simulink model "ap_12BAdapted_with_contracts_AutoPilot"  (R2017b)
settings: Solver=FixedStepDiscrete  StartTime=0.0  StopTime=500  FixedStep=Ts  RelTol=1e-3  EnableMultiTasking=on
undefined symbols (not defined in the file): beaver_b, beaver_c, beaver_mass, beaver_S, Cl0, Cl_alpha2_dpt, Cl_beta, Cl_da, Cl_da_alpha, Cl_dr, Cl_p, Cl_r, Cm0, Cm_alpha, Cm_alpha2, Cm_beta2, Cm_de, Cm_df, Cm_dpt, Cm_q, Cm_r, Cn0, Cn_beta, Cn_beta3, Cn_da, Cn_dpt3, Cn_dr, Cn_p, Cn_q, Cn_r, contractAfterSimulation, contractBeforeSimulation, ContractBlock, ContractEnsureBlock, ContractGuaranteeBlock, ContractModeBlock, ContractRequireBlock, ContractValidatorBlock, Cx0, Cx_alpha, Cx_alpha2, Cx_alpha3, Cx_df, Cx_df_alpha, Cx_dpt, Cx_dpt2_alpha, Cx_dr, Cx_q, Cy0, Cy_beta, Cy_da, Cy_dr, Cy_dr_alpha, Cy_p, Cy_r, Cz0, Cz_alpha, Cz_alpha3, Cz_de, Cz_de_beta ... (+32)
libraries: simulink x10, cocosimLibs x3
(part 1 of 4)
settings Model: Creator=elliocm  LastModifiedBy=hbourbou
settings DataIOCC: LimitDataPoints=on  SaveFormat=Array
settings OptimizationCC: ExpressionDepthLimit=2147483647  LifeSpan=inf
settings DebuggingCC: SolverPrmCheckMsg=warning  StateNameClashWarn=warning  SFUnexpectedBacktrackingDiag=warning  SFNoUnconditionalDefaultTransitionDiag=warning  SFExecutionAtInitializationDiag=none
settings HardwareCC: ProdBitPerPointer=32  ProdBitPerSizeT=32  ProdBitPerPtrDiffT=32  ProdLargestAtomicFloat=None  ProdIntDivRoundTo=Undefined  ProdEndianess=Unspecified  ProdWordSize=32  ProdHWDeviceType=32-bit Generic
settings ModelReferenceCC: PropagateSignalLabelsOutOfModel=off
settings CodeAppCC: StateflowObjectComments=on
settings GRTTargetCC: TargetLangStandard=C89/C90 (ANSI)  GeneratePreprocessorConditionals=Disable all
settings ConfigComp: CovMetricSettings=dw  CovHtmlReporting=on  CovSaveCumulativeToWorkspaceVar=on  CovSaveSingleToWorkspaceVar=on  CovExternalEMLEnable=off

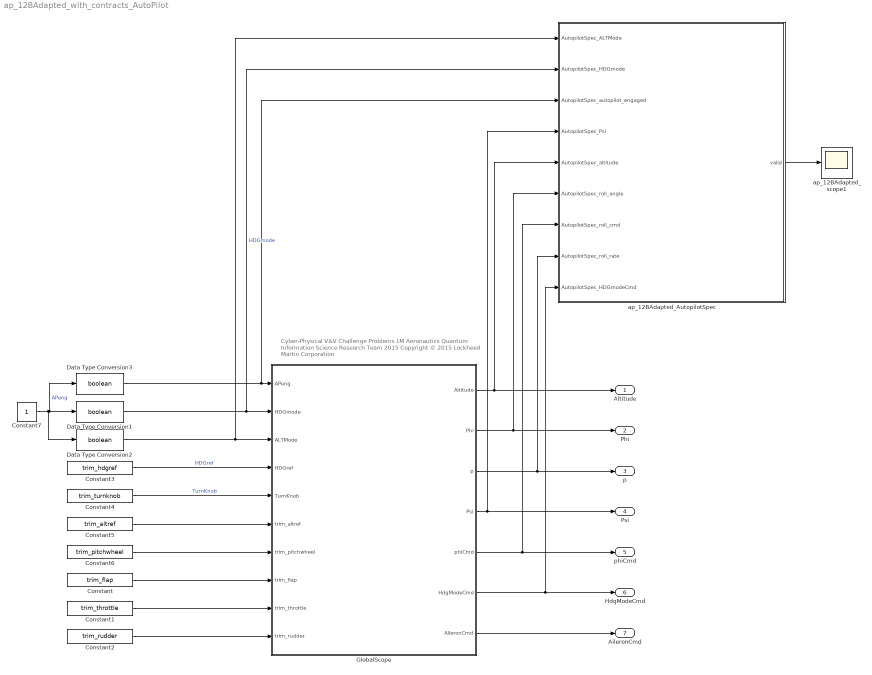
== system ap_12BAdapted_with_contracts_AutoPilot ==
  note: Cyber-Physical V&V Challenge Problems
      | LM Aeronautics Quantum Information Science Research Team 2015
      | Copyright © 2015 Lockheed Martin Corporation
  Constant : Constant  Value=trim_flap
  Constant1 : Constant  Value=trim_throttle
  Constant2 : Constant  Value=trim_rudder
  Constant3 : Constant  Value=trim_hdgref
  Constant4 : Constant  Value=trim_turnknob
  Constant5 : Constant  Value=trim_altref
  Constant6 : Constant  Value=trim_pitchwheel
  Constant7 : Constant
  Data Type Conversion1 : DataTypeConversion  OutDataTypeStr=boolean
  Data Type Conversion2 : DataTypeConversion  OutDataTypeStr=boolean
  Data Type Conversion3 : DataTypeConversion  OutDataTypeStr=boolean
  GlobalScope : Subsystem
  ap_12BAdapted_AutopilotSpec : Subsystem  mask(ContractBlock){ContractBlockType=ContractBlock}
      mask init:
      | set_param(gcb, 'LinkStatus', 'none');
      mask DialogControl DescTextVar Prompt: Contract block
      mask Display:
      | text(0.5, 0.5, '{\bf\fontsize{20}Contract}', 'hor', 'center', 'texmode','on');
      | blocks = find_system(gcb, 'LookUnderMasks','all', 'SearchDepth',1,'BlockType','Inport');
      | for i = 1 : length(blocks)
      |     blockName = get_param(blocks(i), 'Name');
      |     [path, blockName] = fileparts(char(blockName));
      |     port_label('input', i, blockName);
      | end
      | 
      | blocks = find_system(gcb, 'LookUnderMasks','all', 'SearchDepth',1,'BlockType','Outport');
      | for i = 1 : length(blocks)
      |     blockName = get_param(blocks(i), 'Name');
      |     [path, blockName] = fileparts(char(blockName));
      |     port_label('output', i, blockName);
      | end
  ap_12BAdapted_scope1 : Scope
  Altitude : Outport  VectorParamsAs1DForOutWhenUnconnected=off
  Phi : Outport  Port=2  VectorParamsAs1DForOutWhenUnconnected=off
  p : Outport  Port=3  VectorParamsAs1DForOutWhenUnconnected=off
  Psi : Outport  Port=4  VectorParamsAs1DForOutWhenUnconnected=off
  phiCmd : Outport  Port=5  VectorParamsAs1DForOutWhenUnconnected=off
  HdgModeCmd : Outport  Port=6  VectorParamsAs1DForOutWhenUnconnected=off
  AileronCmd : Outport  Port=7  VectorParamsAs1DForOutWhenUnconnected=off
  wires:
  Constant7/1 -> Data Type Conversion2/1, Data Type Conversion3/1, Data Type Conversion1/1  "APeng"
  Data Type Conversion3/1 -> ap_12BAdapted_AutopilotSpec/3(AutopilotSpec_autopilot_engaged), GlobalScope/1(APeng)
  Data Type Conversion1/1 -> ap_12BAdapted_AutopilotSpec/2(AutopilotSpec_HDGmode), GlobalScope/2(HDGmode)  "HDGmode"
  Data Type Conversion2/1 -> ap_12BAdapted_AutopilotSpec/1(AutopilotSpec_ALTMode), GlobalScope/3(ALTMode)
  Constant3/1 -> GlobalScope/4(HDGref)  "HDGref"
  Constant4/1 -> GlobalScope/5(TurnKnob)  "TurnKnob"
  Constant5/1 -> GlobalScope/6(trim_altref)
  Constant6/1 -> GlobalScope/7(trim_pitchwheel)
  GlobalScope/1(Altitude) -> ap_12BAdapted_AutopilotSpec/5(AutopilotSpec_altitude), Altitude/1
  Constant/1 -> GlobalScope/8(trim_flap)
  Constant2/1 -> GlobalScope/10(trim_rudder)
  Constant1/1 -> GlobalScope/9(trim_throttle)
  GlobalScope/6(HdgModeCmd) -> ap_12BAdapted_AutopilotSpec/9(AutopilotSpec_HDGmodeCmd), HdgModeCmd/1
  GlobalScope/5(phiCmd) -> ap_12BAdapted_AutopilotSpec/7(AutopilotSpec_roll_cmd), phiCmd/1
  GlobalScope/7(AileronCmd) -> AileronCmd/1
  GlobalScope/4(Psi) -> ap_12BAdapted_AutopilotSpec/4(AutopilotSpec_Psi), Psi/1
  GlobalScope/3(p) -> ap_12BAdapted_AutopilotSpec/8(AutopilotSpec_roll_rate), p/1
  GlobalScope/2(Phi) -> ap_12BAdapted_AutopilotSpec/6(AutopilotSpec_roll_angle), Phi/1
  ap_12BAdapted_AutopilotSpec/1(valid) -> ap_12BAdapted_scope1/1

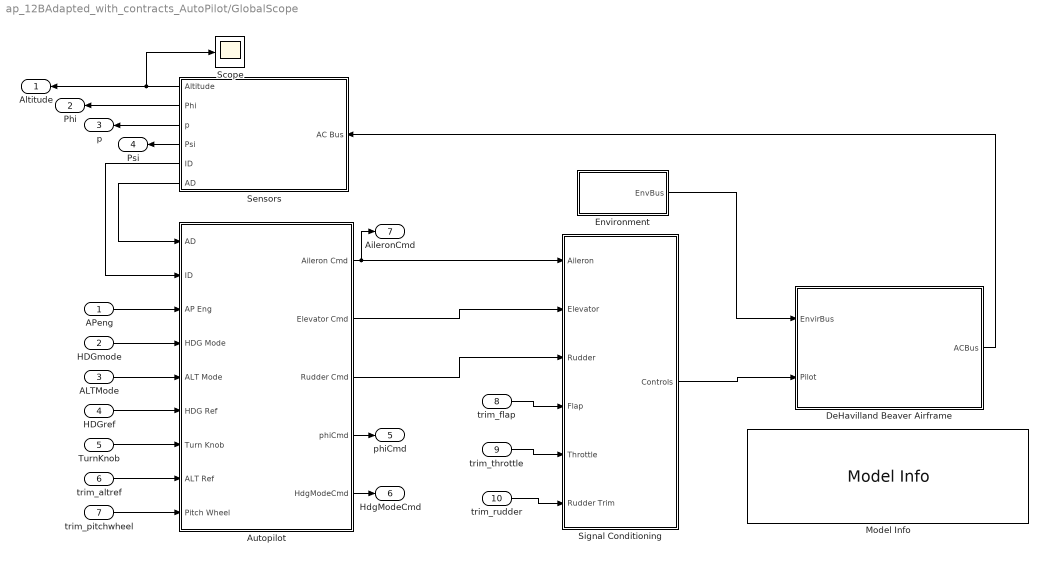
== system ap_12BAdapted_with_contracts_AutoPilot/GlobalScope ==
  APeng : Inport
  HDGmode : Inport  Port=2
  ALTMode : Inport  Port=3
  HDGref : Inport  Port=4
  TurnKnob : Inport  Port=5
  trim_altref : Inport  Port=6
  trim_pitchwheel : Inport  Port=7
  trim_flap : Inport  Port=8
  trim_throttle : Inport  Port=9
  trim_rudder : Inport  Port=10
  Autopilot : Subsystem  TreatAsAtomicUnit=on
  DeHavilland Beaver Airframe : Subsystem  TreatAsAtomicUnit=on
      mask Display:
      | %image(imread('asbbeaver.jpg'))
      | image(imread('asbbeaver.png'))
  Environment : Subsystem
  Model Info : simulink/Model-Wide Utilities/Model Info  Frame=on  DisplayStringWithTags=|  HorizontalTextAlignment=Center  LeftAlignmentValue=0.5
      | DeHavilland Beaver model 
      | originally based on work created by
      | Marc Rauw for Delft University of Technology,  
      | http://www.dutchroll.com
      | and subsequently modified by the Mathworks
      | http://www.mathworks.com/matlabcentral/fileexchange/
  Scope : Scope
  Sensors : Subsystem
  Signal Conditioning : Subsystem  TreatAsAtomicUnit=on
  Altitude : Outport  VectorParamsAs1DForOutWhenUnconnected=off
  Phi : Outport  Port=2  VectorParamsAs1DForOutWhenUnconnected=off
  p : Outport  Port=3  VectorParamsAs1DForOutWhenUnconnected=off
  Psi : Outport  Port=4  VectorParamsAs1DForOutWhenUnconnected=off
  phiCmd : Outport  Port=5  VectorParamsAs1DForOutWhenUnconnected=off
  HdgModeCmd : Outport  Port=6  VectorParamsAs1DForOutWhenUnconnected=off
  AileronCmd : Outport  Port=7  VectorParamsAs1DForOutWhenUnconnected=off
  wires:
  Autopilot/1(Aileron Cmd) -> AileronCmd/1, Signal Conditioning/1(Aileron)
  Sensors/1(Altitude) -> Altitude/1, Scope/1
  trim_altref/1 -> Autopilot/8(ALT Ref)
  Autopilot/3(Rudder Cmd) -> Signal Conditioning/3(Rudder)
  ALTMode/1 -> Autopilot/5(ALT Mode)
  TurnKnob/1 -> Autopilot/7(Turn Knob)
  trim_throttle/1 -> Signal Conditioning/5(Throttle)
  trim_rudder/1 -> Signal Conditioning/6(Rudder Trim)
  trim_flap/1 -> Signal Conditioning/4(Flap)
  trim_pitchwheel/1 -> Autopilot/9(Pitch Wheel)
  APeng/1 -> Autopilot/3(AP Eng)
  Environment/1(EnvBus) -> DeHavilland Beaver Airframe/1(EnvirBus)
  Autopilot/2(Elevator Cmd) -> Signal Conditioning/2(Elevator)
  DeHavilland Beaver Airframe/1(ACBus) -> Sensors/1(AC Bus)
  HDGmode/1 -> Autopilot/4(HDG Mode)
  HDGref/1 -> Autopilot/6(HDG Ref)
  Sensors/6(AD) -> Autopilot/1(AD)
  Sensors/5(ID) -> Autopilot/2(ID)
  Autopilot/4(phiCmd) -> phiCmd/1
  Sensors/2(Phi) -> Phi/1
  Sensors/3(p) -> p/1
  Autopilot/5(HdgModeCmd) -> HdgModeCmd/1
  Sensors/4(Psi) -> Psi/1
  Signal Conditioning/1(Controls) -> DeHavilland Beaver Airframe/2(Pilot)

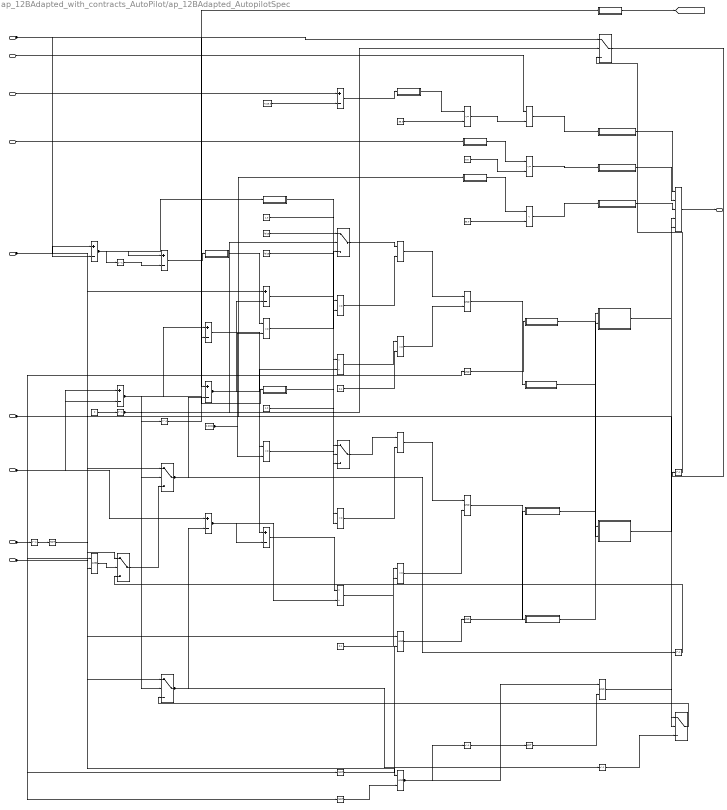
== system ap_12BAdapted_with_contracts_AutoPilot/ap_12BAdapted_AutopilotSpec ==
  AutopilotSpec_ALTMode : Inport  OutDataTypeStr=boolean
  AutopilotSpec_HDGmode : Inport  Port=2  OutDataTypeStr=boolean
  AutopilotSpec_autopilot_engaged : Inport  Port=3  OutDataTypeStr=boolean
  AutopilotSpec_Psi : Inport  Port=4  OutDataTypeStr=double
  AutopilotSpec_altitude : Inport  Port=5  OutDataTypeStr=double
  AutopilotSpec_roll_angle : Inport  Port=6  OutDataTypeStr=double
  AutopilotSpec_roll_cmd : Inport  Port=7  OutDataTypeStr=double
  AutopilotSpec_roll_rate : Inport  Port=8  OutDataTypeStr=double
  AutopilotSpec_HDGmodeCmd : Inport  Port=9  OutDataTypeStr=double
  AP-000 : Subsystem  mask(ContractGuaranteeBlock){ContractBlockType=ContractGuaranteeBlock}
      mask init:
      | set_param(gcb, 'LinkStatus', 'none');
      mask DialogControl DescTextVar Prompt: Guarantee block
  AP-005 : Subsystem  mask(ContractGuaranteeBlock){ContractBlockType=ContractGuaranteeBlock}
      mask init:
      | set_param(gcb, 'LinkStatus', 'none');
      mask DialogControl DescTextVar Prompt: Guarantee block
  AP-006 : Subsystem  mask(ContractGuaranteeBlock){ContractBlockType=ContractGuaranteeBlock}
      mask init:
      | set_param(gcb, 'LinkStatus', 'none');
      mask DialogControl DescTextVar Prompt: Guarantee block
  Arrow_xxAutopilotSpec_9_ni_0 : Delay  DelayLength=1  InitialCondition=1
  PRE_xxAutopilotSpec_{10,13,16,20,25,28,31} (7 alike) : Delay  DelayLength=1  InitialCondition=0
  abs_real_call : Subsystem
  abs_real_call1 : Subsystem
  abs_real_call11 : Subsystem
  abs_real_call111 : Subsystem
  abs_real_call1111 : Subsystem
  abs_real_call11111 : Subsystem
  abs_real_call111111 : Subsystem
  branch_10_IF : Switch  Criteria=u2 ~= 0
  branch_11_IF : Switch  Criteria=u2 ~= 0
  branch_12_IF : Switch  Criteria=u2 ~= 0
  branch_13_IF : Switch  Criteria=u2 ~= 0
  branch_14_IF : Switch  Criteria=u2 ~= 0
  branch_15_IF : Switch  Criteria=u2 ~= 0
  branch_9_IF : Switch  Criteria=u2 ~= 0
  hdg_err_operator : Sum  Inputs=+-  OutDataTypeStr=double
  hdg_mode : Subsystem  mask(ContractModeBlock){ContractBlockType=ContractModeBlock}
      mask init:
      | set_param(gcb, 'LinkStatus', 'none');
      mask DialogControl DescTextVar Prompt: Mode block
  hdg_mode_ensure : Subsystem  mask(ContractEnsureBlock){ContractBlockType=ContractEnsureBlock}
      mask init:
      | set_param(gcb, 'LinkStatus', 'none');
      mask DialogControl DescTextVar Prompt: Ensure block
  hdg_mode_ensure_cond : Logic  AllPortsSameDT=off  OutDataTypeStr=boolean
  hdg_mode_require : Subsystem  mask(ContractRequireBlock){ContractBlockType=ContractRequireBlock}
      mask init:
      | set_param(gcb, 'LinkStatus', 'none');
      mask DialogControl DescTextVar Prompt: Require block
  hdg_mode_require_cond : Logic  Inputs=1  AllPortsSameDT=off  OutDataTypeStr=boolean
  hdg_overshoot_operator : Product  Inputs=*/  OutDataTypeStr=double
  hdg_step_operator : Sum  Inputs=+-  OutDataTypeStr=double
  overshoot_operator : Product  Inputs=*/  OutDataTypeStr=double
  rollHoldMode_operator : Logic  AllPortsSameDT=off  OutDataTypeStr=boolean
  roll_err_operator : Sum  Inputs=+-  OutDataTypeStr=double
  roll_hold_mode : Subsystem  mask(ContractModeBlock){ContractBlockType=ContractModeBlock}
      mask init:
      | set_param(gcb, 'LinkStatus', 'none');
      mask DialogControl DescTextVar Prompt: Mode block
  roll_hold_mode_ensure : Subsystem  mask(ContractEnsureBlock){ContractBlockType=ContractEnsureBlock}
      mask init:
      | set_param(gcb, 'LinkStatus', 'none');
      mask DialogControl DescTextVar Prompt: Ensure block
  roll_hold_mode_ensure_cond : Logic  AllPortsSameDT=off  OutDataTypeStr=boolean
  roll_hold_mode_require : Subsystem  mask(ContractRequireBlock){ContractBlockType=ContractRequireBlock}
      mask init:
      | set_param(gcb, 'LinkStatus', 'none');
      mask DialogControl DescTextVar Prompt: Require block
  roll_hold_mode_require_cond : Logic  Inputs=1  AllPortsSameDT=off  OutDataTypeStr=boolean
  spec219_operator : Logic  AllPortsSameDT=off  OutDataTypeStr=boolean
  spec228_operator : cocosimLibs/Implies  SystemSampleTime=-1  Latency=0  AutoFrameSizeCalculation=off
  spec233_operator : RelationalOperator  Operator=<=  OutDataTypeStr=boolean  RndMeth=Simplest
  spec233_rhs_2 : Constant  Value=0.1  OutDataTypeStr=double
  spec244_operator : cocosimLibs/Implies  SystemSampleTime=-1  Latency=0  AutoFrameSizeCalculation=off
  spec249_operator : RelationalOperator  Operator=<=  OutDataTypeStr=boolean  RndMeth=Simplest
  spec249_rhs_2 : Constant  Value=0.1  OutDataTypeStr=double
  spec263_operator : cocosimLibs/Implies  SystemSampleTime=-1  Latency=0  AutoFrameSizeCalculation=off
  spec268_operator : RelationalOperator  Operator=<=  OutDataTypeStr=boolean  RndMeth=Simplest
  spec268_rhs_2 : Constant  Value=6.6  OutDataTypeStr=double
  spec273_operator : RelationalOperator  Operator=<  OutDataTypeStr=boolean  RndMeth=Simplest
  spec273_rhs_2 : Constant  Value=33.0  OutDataTypeStr=double
  step_operator : Sum  Inputs=+-  OutDataTypeStr=double
  validator : M-S-Function  LoadFcn=saveValidatorParameters(gcb);  InitFcn=contractBeforeSimulation();  StopFcn=contractAfterSimulation();  FunctionName=contract  mask(ContractValidatorBlock){assumePorts=0, guaranteePorts=3, modePorts=2, ContractBlockType=ContractValidatorBlock, createInportsCheckbox=off}
      mask prompts: assumePorts "Assume ports     :"; guaranteePorts "Guarantee ports :"; modePorts "Mode ports        :"; createInportsCheckbox "Create inports and connect them automatically"
      mask init:
      | set_param(gcb,'LinkStatus','none');
      | contract_callback('inputs_callback',gcb);
      mask DialogControl DescTextVar Prompt: The validator block implements the following logic: <br> <br> <b>Sofar</b>(assume<sub>1</sub> <b>&#8743;</b> assume<sub>2</sub> <b>&#8743;</b> ... assume<sub>k</sub>) <b>&rarr;</b> (guarantee<sub>1</sub> <b>&#8743;</b> guarantee<sub>2</sub> <b>&#8743;</b> ... guarantee<sub>m</sub> <b>&#8743;</b>  mode<sub>1</sub> <b>&#8743;</b> mode<sub>2</sub> <b>&#8743;</b> ... <b>&#8743;</b> mode<sub>n</sub> )<br> where mode<sub>i</sub> = require<sub>i</sub> <b>&rarr;</b> ensure<sub>i</sub>
      mask Display:
      | color('black');
      | port_label('input',1,'guarantee');
      | port_label('input',2,'guarantee');
      | port_label('input',3,'guarantee');
      | port_label('input',4,'mode');
      | port_label('input',5,'mode');
      | port_label('output',1,'valid');
  xxAutopilotSpec_11_operator : Logic  Operator=NOT  AllPortsSameDT=off  OutDataTypeStr=boolean
  xxAutopilotSpec_12_operator : Logic  AllPortsSameDT=off  OutDataTypeStr=boolean
  xxAutopilotSpec_15_operator : Logic  Operator=NOT  AllPortsSameDT=off  OutDataTypeStr=boolean
  xxAutopilotSpec_17_operator : Sum  Inputs=+-  OutDataTypeStr=double
  xxAutopilotSpec_18_operator : RelationalOperator  Operator=<=  OutDataTypeStr=boolean  RndMeth=Simplest
  xxAutopilotSpec_19_rhs1 : Constant  Value=false  OutDataTypeStr=boolean
  xxAutopilotSpec_1_operator : RelationalOperator  Operator=<=  OutDataTypeStr=boolean  RndMeth=Simplest
  xxAutopilotSpec_1_rhs_2 : Constant  Value=35.0  OutDataTypeStr=double
  xxAutopilotSpec_21_operator : Sum  Inputs=+-  OutDataTypeStr=double
  xxAutopilotSpec_23_operator : RelationalOperator  Operator=<=  OutDataTypeStr=boolean  RndMeth=Simplest
  xxAutopilotSpec_24_rhs1 : Constant  Value=false  OutDataTypeStr=boolean
  xxAutopilotSpec_27_operator : Sum  Inputs=+-  OutDataTypeStr=double
  xxAutopilotSpec_29_operator : Logic  Operator=NOT  AllPortsSameDT=off  OutDataTypeStr=boolean
  xxAutopilotSpec_30_operator : Logic  AllPortsSameDT=off  OutDataTypeStr=boolean
  xxAutopilotSpec_33_rhs : Constant  Value=7225.0  OutDataTypeStr=double
  xxAutopilotSpec_34_operator : Sum  Inputs=+-  OutDataTypeStr=double
  xxAutopilotSpec_3_operator : RelationalOperator  Operator=<=  OutDataTypeStr=boolean  RndMeth=Simplest
  xxAutopilotSpec_3_rhs_2 : Constant  Value=1.0  OutDataTypeStr=double
  xxAutopilotSpec_4_operator : Logic  Operator=NOT  AllPortsSameDT=off  OutDataTypeStr=boolean
  xxAutopilotSpec_6_operator : RelationalOperator  Operator=<=  OutDataTypeStr=boolean  RndMeth=Simplest
  xxAutopilotSpec_6_rhs_2 : Constant  Value=1.0  OutDataTypeStr=double
  xxAutopilotSpec_7_rhs : Constant  Value=0.0001  OutDataTypeStr=double
  xxAutopilotSpec_8_operator : Sum  Inputs=+-  OutDataTypeStr=double
  xxAutopilotSpec_9_ni_0_init : Constant  Value=0  OutDataTypeStr=boolean
  valid : Outport
  wires:
  validator/1 -> valid/1
  xxAutopilotSpec_6_rhs_2/1 -> xxAutopilotSpec_6_operator/2
  abs_real_call11111/1(abs_real_y) -> xxAutopilotSpec_6_operator/1
  xxAutopilotSpec_3_rhs_2/1 -> xxAutopilotSpec_3_operator/2
  abs_real_call1111/1(abs_real_y) -> xxAutopilotSpec_3_operator/1
  xxAutopilotSpec_33_rhs/1 -> xxAutopilotSpec_34_operator/2
  AutopilotSpec_altitude/1 -> xxAutopilotSpec_34_operator/1
  xxAutopilotSpec_29_operator/1 -> xxAutopilotSpec_30_operator/2
  PRE_xxAutopilotSpec_28/1 -> xxAutopilotSpec_29_operator/1
  abs_real_call111/1(abs_real_y) -> xxAutopilotSpec_23_operator/1
  PRE_xxAutopilotSpec_20/1 -> xxAutopilotSpec_21_operator/2
  xxAutopilotSpec_1_rhs_2/1 -> xxAutopilotSpec_1_operator/2
  abs_real_call11/1(abs_real_y) -> xxAutopilotSpec_1_operator/1
  xxAutopilotSpec_17_operator/1 -> xxAutopilotSpec_18_operator/1
  PRE_xxAutopilotSpec_16/1 -> xxAutopilotSpec_17_operator/2
  xxAutopilotSpec_11_operator/1 -> xxAutopilotSpec_12_operator/2
  PRE_xxAutopilotSpec_10/1 -> xxAutopilotSpec_11_operator/1
  hdg_mode/1(mode) -> validator/5
  roll_hold_mode/1(mode) -> validator/4
  AP-006/1(guarantee) -> validator/3
  AP-005/1(guarantee) -> validator/2
  AP-000/1(guarantee) -> validator/1
  spec273_rhs_2/1 -> spec273_operator/2
  abs_real_call/1(abs_real_y) -> spec273_operator/1
  spec268_rhs_2/1 -> spec268_operator/2
  abs_real_call1/1(abs_real_y) -> spec268_operator/1
  xxAutopilotSpec_1_operator/1 -> spec263_operator/2
  AutopilotSpec_ALTMode/1 -> spec263_operator/1
  spec249_rhs_2/1 -> spec249_operator/2
  hdg_overshoot_operator/1 -> spec249_operator/1
  xxAutopilotSpec_3_operator/1 -> spec244_operator/2
  branch_14_IF/1 -> spec244_operator/1
  spec233_rhs_2/1 -> spec233_operator/2
  overshoot_operator/1 -> spec233_operator/1
  xxAutopilotSpec_6_operator/1 -> spec228_operator/2
  branch_11_IF/1 -> spec228_operator/1
  xxAutopilotSpec_4_operator/1 -> spec219_operator/2
  spec219_operator/1 -> roll_hold_mode_require_cond/1
  roll_hold_mode_require_cond/1 -> roll_hold_mode_require/1(In1)
  spec233_operator/1 -> roll_hold_mode_ensure_cond/2
  spec228_operator/1 -> roll_hold_mode_ensure_cond/1
  roll_hold_mode_ensure_cond/1 -> roll_hold_mode_ensure/1(In1)
  roll_hold_mode_ensure/1(ensure) -> roll_hold_mode/2(ensure)
  roll_hold_mode_require/1(require) -> roll_hold_mode/1(require)
  xxAutopilotSpec_15_operator/1 -> rollHoldMode_operator/2
  xxAutopilotSpec_8_operator/1 -> overshoot_operator/1
  xxAutopilotSpec_27_operator/1 -> hdg_overshoot_operator/1
  hdg_mode_require_cond/1 -> hdg_mode_require/1(In1)
  spec249_operator/1 -> hdg_mode_ensure_cond/2
  spec244_operator/1 -> hdg_mode_ensure_cond/1
  hdg_mode_ensure_cond/1 -> hdg_mode_ensure/1(In1)
  hdg_mode_ensure/1(ensure) -> hdg_mode/2(ensure)
  hdg_mode_require/1(require) -> hdg_mode/1(require)
  branch_10_IF/1 -> branch_9_IF/3
  PRE_xxAutopilotSpec_25/1 -> branch_15_IF/3
  xxAutopilotSpec_23_operator/1 -> branch_14_IF/3
  xxAutopilotSpec_24_rhs1/1 -> branch_14_IF/1
  PRE_xxAutopilotSpec_31/1 -> branch_13_IF/3
  xxAutopilotSpec_30_operator/1 -> branch_13_IF/2
  branch_13_IF/1 -> branch_12_IF/3
  xxAutopilotSpec_18_operator/1 -> branch_11_IF/3
  xxAutopilotSpec_19_rhs1/1 -> branch_11_IF/1
  PRE_xxAutopilotSpec_13/1 -> branch_10_IF/3
  xxAutopilotSpec_12_operator/1 -> branch_10_IF/2
  abs_real_call111111/1(abs_real_y) -> [AutopilotSpec_abs_roller_err]
  xxAutopilotSpec_21_operator/1 -> abs_real_call111/1(abs_real_x)
  xxAutopilotSpec_34_operator/1 -> abs_real_call11/1(abs_real_x)
  AutopilotSpec_roll_rate/1 -> abs_real_call1/1(abs_real_x)
  branch_15_IF/1 -> PRE_xxAutopilotSpec_25/1
  xxAutopilotSpec_9_ni_0_init/1 -> Arrow_xxAutopilotSpec_9_ni_0/1
  spec273_operator/1 -> AP-006/1(In1)
  spec268_operator/1 -> AP-005/1(In1)
  spec263_operator/1 -> AP-000/1(In1)
  AutopilotSpec_HDGmode/1 -> xxAutopilotSpec_4_operator/1, xxAutopilotSpec_30_operator/1, xxAutopilotSpec_15_operator/1, hdg_mode_require_cond/1, PRE_xxAutopilotSpec_28/1
  rollHoldMode_operator/1 -> xxAutopilotSpec_12_operator/1, PRE_xxAutopilotSpec_10/1
  AutopilotSpec_HDGmodeCmd/1 -> hdg_step_operator/1, hdg_err_operator/2, branch_15_IF/1
  roll_err_operator/1 -> xxAutopilotSpec_17_operator/1, abs_real_call111111/1(abs_real_x), abs_real_call11111/1(abs_real_x), PRE_xxAutopilotSpec_16/1
  step_operator/1 -> xxAutopilotSpec_8_operator/2, overshoot_operator/2
  hdg_err_operator/1 -> xxAutopilotSpec_21_operator/1, abs_real_call1111/1(abs_real_x), PRE_xxAutopilotSpec_20/1
  hdg_step_operator/1 -> xxAutopilotSpec_27_operator/2, hdg_overshoot_operator/2
  branch_12_IF/1 -> hdg_step_operator/2, PRE_xxAutopilotSpec_31/1
  AutopilotSpec_Psi/1 -> xxAutopilotSpec_27_operator/1, hdg_err_operator/1, branch_13_IF/1, branch_12_IF/1
  AutopilotSpec_roll_angle/1 -> xxAutopilotSpec_8_operator/1, roll_err_operator/1, branch_9_IF/1, branch_10_IF/1, abs_real_call/1(abs_real_x)
  Arrow_xxAutopilotSpec_9_ni_0/1 -> branch_9_IF/2, branch_15_IF/2, branch_14_IF/2, branch_12_IF/2, branch_11_IF/2
  xxAutopilotSpec_7_rhs/1 -> xxAutopilotSpec_23_operator/2, xxAutopilotSpec_18_operator/2
  AutopilotSpec_roll_cmd/1 -> step_operator/1, roll_err_operator/2
  branch_9_IF/1 -> step_operator/2, PRE_xxAutopilotSpec_13/1
  AutopilotSpec_autopilot_engaged/1 -> spec219_operator/1, rollHoldMode_operator/1

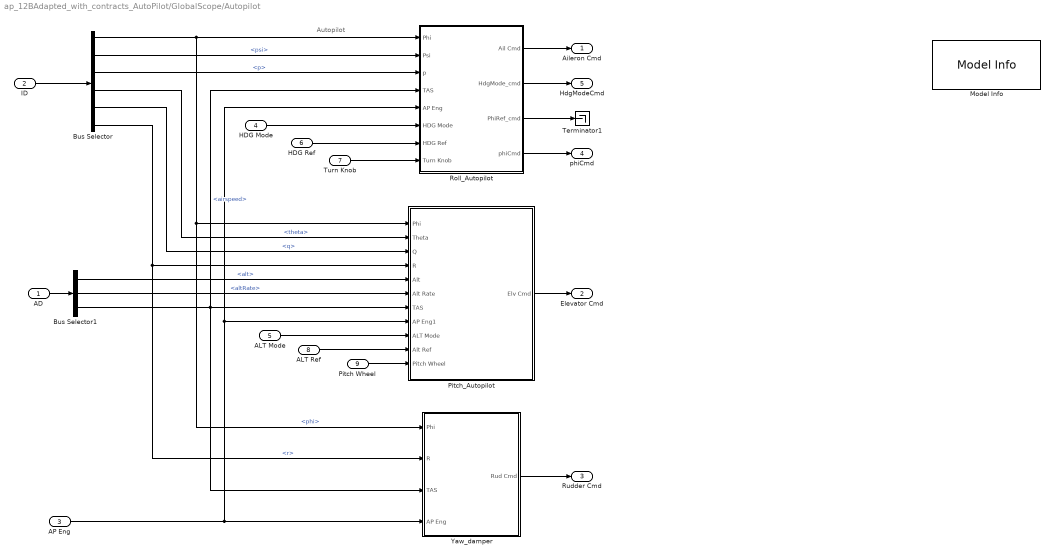
== system ap_12BAdapted_with_contracts_AutoPilot/GlobalScope/Autopilot ==
  note: Autopilot
  AD : Inport
  ID : Inport  Port=2
  AP Eng : Inport  Port=3  OutMin=0  OutMax=1  OutDataTypeStr=boolean  PortDimensions=1
  HDG Mode : Inport  Port=4  OutMin=0  OutMax=1  OutDataTypeStr=boolean  PortDimensions=1
  ALT Mode : Inport  Port=5  OutMin=0  OutMax=1  OutDataTypeStr=boolean  PortDimensions=1
  HDG Ref : Inport  Port=6  OutMin=-180  OutMax=180  OutDataTypeStr=double  PortDimensions=1
  Turn Knob : Inport  Port=7  OutMin=-45  OutMax=45  OutDataTypeStr=double  PortDimensions=1
  ALT Ref : Inport  Port=8  OutMin=0  OutMax=65000  OutDataTypeStr=double  PortDimensions=1
  Pitch Wheel : Inport  Port=9  OutMin=-30  OutMax=30  OutDataTypeStr=double  PortDimensions=1
  Bus Selector : BusSelector  OutputSignals=phi,psi,p,theta,q,r
  Bus Selector1 : BusSelector  OutputSignals=alt,altRate,airspeed
  Model Info : simulink/Model-Wide Utilities/Model Info  Frame=on  DisplayStringWithTags=|  HorizontalTextAlignment=Left  LeftAlignmentValue=0.02
      | Autopilot
      | Author: %<LastModifiedBy>
      | Date: %<LastModificationDate>
      | Model Version: %<ModelVersion>
  Pitch_Autopilot : Subsystem
  Roll_Autopilot : Subsystem
  Terminator1 : Terminator
  Yaw_damper : Subsystem
  Aileron Cmd : Outport  OutDataTypeStr=double  PortDimensions=1  SampleTime=[0.025000000000000001,0]  VectorParamsAs1DForOutWhenUnconnected=off
  Elevator Cmd : Outport  Port=2  OutDataTypeStr=double  PortDimensions=1  SampleTime=[0.025000000000000001,0]  VectorParamsAs1DForOutWhenUnconnected=off
  Rudder Cmd : Outport  Port=3  OutDataTypeStr=double  PortDimensions=1  SampleTime=[0.025000000000000001,0]  VectorParamsAs1DForOutWhenUnconnected=off
  phiCmd : Outport  Port=4  VectorParamsAs1DForOutWhenUnconnected=off
  HdgModeCmd : Outport  Port=5  VectorParamsAs1DForOutWhenUnconnected=off
  wires:
  Roll_Autopilot/1(Ail Cmd) -> Aileron Cmd/1
  HDG Ref/1 -> Roll_Autopilot/7(HDG Ref)
  Bus Selector/6 -> Yaw_damper/2(R), Pitch_Autopilot/4(R)  "<r>"
  Bus Selector1/3 -> Yaw_damper/3(TAS), Roll_Autopilot/4(TAS), Pitch_Autopilot/7(TAS)  "<airspeed>"
  HDG Mode/1 -> Roll_Autopilot/6(HDG Mode)
  Pitch_Autopilot/1(Elv Cmd) -> Elevator Cmd/1
  ALT Mode/1 -> Pitch_Autopilot/9(ALT Mode)
  ALT Ref/1 -> Pitch_Autopilot/10(Alt Ref)
  Pitch Wheel/1 -> Pitch_Autopilot/11("Pitch Wheel ")
  Bus Selector1/1 -> Pitch_Autopilot/5(Alt)  "<alt>"
  Yaw_damper/1(Rud Cmd) -> Rudder Cmd/1
  AP Eng/1 -> Yaw_damper/4(AP Eng), Roll_Autopilot/5(AP Eng), Pitch_Autopilot/8(AP Eng1)
  Bus Selector/3 -> Roll_Autopilot/3(p)  "<p>"
  Turn Knob/1 -> Roll_Autopilot/8(Turn Knob)
  Bus Selector/1 -> Pitch_Autopilot/1(Phi), Yaw_damper/1(Phi), Roll_Autopilot/1(Phi)  "<phi>"
  Bus Selector/2 -> Roll_Autopilot/2(Psi)  "<psi>"
  Bus Selector/5 -> Pitch_Autopilot/3(Q)  "<q>"
  Bus Selector/4 -> Pitch_Autopilot/2(Theta)  "<theta>"
  ID/1 -> Bus Selector/1
  AD/1 -> Bus Selector1/1
  Bus Selector1/2 -> Pitch_Autopilot/6(Alt Rate)  "<altRate>"
  Roll_Autopilot/4(phiCmd) -> phiCmd/1
  Roll_Autopilot/2(HdgMode_cmd) -> HdgModeCmd/1
  Roll_Autopilot/3(PhiRef_cmd) -> Terminator1/1

== system ap_12BAdapted_with_contracts_AutoPilot/GlobalScope/DeHavilland Beaver Airframe ==
  note: DeHavilland Beaver Airframe
  EnvirBus : Inport
  Pilot : Inport  Port=2
  Aircraft Dynamics : Subsystem
  Calculate Parameters : Subsystem
  ACBus : Outport  VectorParamsAs1DForOutWhenUnconnected=off
  wires:
  Pilot/1 -> Aircraft Dynamics/1(Pilot)
  Aircraft Dynamics/1(AC Bus) -> ACBus/1, Calculate Parameters/2(ACBus)
  EnvirBus/1 -> Aircraft Dynamics/2(EnvirBus), Calculate Parameters/1(EnvirBus)
  Calculate Parameters/1(FltParams) -> Aircraft Dynamics/3(FltParams)

== system ap_12BAdapted_with_contracts_AutoPilot/GlobalScope/Environment ==
  note: Environment
  Bus Creator : BusCreator  Inputs=3
  Bus Creator1 : BusCreator  Inputs=2
  Mux : Mux  Inputs=3
  Mux1 : Mux  Inputs=3
  g_mps2 : Constant  Value=9.799
  rho_kgpm3 : Constant  Value=0.9862
  wind_mps : Constant  Value=0
  EnvBus : Outport  VectorParamsAs1DForOutWhenUnconnected=off
  wires:
  g_mps2/1 -> Bus Creator/1  "g"
  Mux1/1 -> Bus Creator1/2  "pqr_wind"
  Mux/1 -> Bus Creator1/1  "uvw_wind"
  Bus Creator1/1 -> Bus Creator/3  "Vwind"
  Bus Creator/1 -> EnvBus/1
  rho_kgpm3/1 -> Bus Creator/2  "rho"
  wind_mps/1 -> Mux1/3, Mux1/2, Mux1/1, Mux/3, Mux/2, Mux/1

== system ap_12BAdapted_with_contracts_AutoPilot/GlobalScope/Sensors ==
  AC Bus : Inport
  Air Data Sensor : Subsystem
  Bus Creator : BusCreator  Inputs=6
  Bus Creator1 : BusCreator  Inputs=5
  Bus Creator2 : BusCreator  Inputs=2
  Display : Display
  Display1 : Display
  Inertial Data Sensor : Subsystem
  Scope : Scope  NumInputPorts=5
  Scope1 : Scope  NumInputPorts=6
  Terminator : Terminator
  Altitude : Outport  VectorParamsAs1DForOutWhenUnconnected=off
  Phi : Outport  Port=2  VectorParamsAs1DForOutWhenUnconnected=off
  p : Outport  Port=3  VectorParamsAs1DForOutWhenUnconnected=off
  Psi : Outport  Port=4  VectorParamsAs1DForOutWhenUnconnected=off
  ID : Outport  Port=5  VectorParamsAs1DForOutWhenUnconnected=off
  AD : Outport  Port=6  VectorParamsAs1DForOutWhenUnconnected=off
  wires:
  AC Bus/1 -> Air Data Sensor/1(AC Bus), Inertial Data Sensor/1(AC Bus)
  Inertial Data Sensor/3(psi) -> Scope1/3, Psi/1, Bus Creator/3  "psi"
  Inertial Data Sensor/2(theta) -> Scope1/2, Bus Creator/2  "theta"
  Inertial Data Sensor/4(p) -> Scope1/4, p/1, Bus Creator/4  "p"
  Inertial Data Sensor/1(phi) -> Scope1/1, Phi/1, Bus Creator/1
  Inertial Data Sensor/5(q) -> Scope1/5, Bus Creator/5  "q"
  Inertial Data Sensor/6(r) -> Scope1/6, Bus Creator/6  "r"
  Bus Creator/1 -> Bus Creator2/1, Display/1, ID/1  "ID"
  Air Data Sensor/1(altRate) -> Scope/1, Bus Creator1/1  "altRate"
  Air Data Sensor/2(alpha) -> Scope/2, Bus Creator1/2  "alpha"
  Air Data Sensor/3(beta) -> Scope/3, Bus Creator1/3  "beta"
  Air Data Sensor/4(airspeed) -> Scope/4, Bus Creator1/4  "airspeed"
  Air Data Sensor/5(alt) -> Scope/5, Altitude/1, Bus Creator1/5  "alt"
  Bus Creator1/1 -> Bus Creator2/2, Display1/1, AD/1  "AD"
  Bus Creator2/1 -> Terminator/1

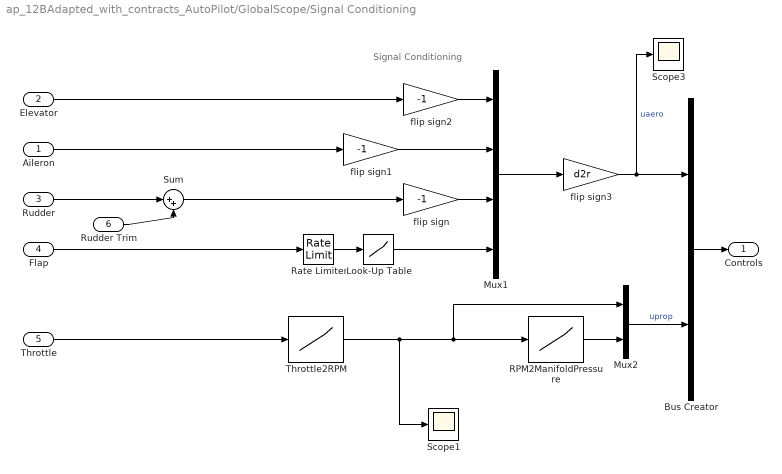
== system ap_12BAdapted_with_contracts_AutoPilot/GlobalScope/Signal Conditioning ==
  note: Signal Conditioning
  Aileron : Inport
  Elevator : Inport  Port=2
  Rudder : Inport  Port=3
  Flap : Inport  Port=4
  Throttle : Inport  Port=5
  Rudder Trim : Inport  Port=6
  Bus Creator : BusCreator  Inputs=2
  Look-Up Table : Lookup_n-D  NumberOfTableDimensions=1  BreakpointsForDimension1=[0:3]  Table=[0 4 10 20]  InternalRulePriority=Speed  SaturateOnIntegerOverflow=on  InputSameDT=on
  Mux1 : Mux
  Mux2 : Mux  Inputs=2
  RPM2ManifoldPressure : Lookup_n-D  NumberOfTableDimensions=1  BreakpointsForDimension1=[0 1800 2300]  IndexSearchMethod=Linear search  BeginIndexSearchUsingPreviousIndexResult=on  Table=[0 22.5735 26]  ExtrapMethod=Clip  InputSameDT=on
  Rate Limiter : RateLimiter  RisingSlewLimit=0.5  FallingSlewLimit=-0.5
  Scope1 : Scope
  Scope3 : Scope
  Sum : Sum  Inputs=|++
  Throttle2RPM : Lookup_n-D  NumberOfTableDimensions=1  BreakpointsForDimension1=(1/6)*(3+([-3:3]))  IndexSearchMethod=Linear search  BeginIndexSearchUsingPreviousIndexResult=on  Table=((1+tanh([-3:3]))/(1+tanh(2.65))-0.0025)*2300  ExtrapMethod=Clip  InputSameDT=on
  flip sign : Gain  Gain=-1  SaturateOnIntegerOverflow=on  OutDataTypeStr=Inherit: Same as input  ParamDataTypeStr=Inherit: Same as input
  flip sign1 : Gain  Gain=-1  SaturateOnIntegerOverflow=on  OutDataTypeStr=Inherit: Same as input  ParamDataTypeStr=Inherit: Same as input
  flip sign2 : Gain  Gain=-1  SaturateOnIntegerOverflow=on  OutDataTypeStr=Inherit: Same as input  ParamDataTypeStr=Inherit: Same as input
  flip sign3 : Gain  Gain=d2r  SaturateOnIntegerOverflow=on  OutDataTypeStr=Inherit: Same as input  ParamDataTypeStr=Inherit: Same as input
  Controls : Outport  VectorParamsAs1DForOutWhenUnconnected=off
  wires:
  Bus Creator/1 -> Controls/1
  Throttle/1 -> Throttle2RPM/1
  Sum/1 -> flip sign/1
  Aileron/1 -> flip sign1/1
  Elevator/1 -> flip sign2/1
  flip sign2/1 -> Mux1/1
  flip sign1/1 -> Mux1/2
  Throttle2RPM/1 -> Scope1/1, RPM2ManifoldPressure/1, Mux2/1
  flip sign/1 -> Mux1/3
  Mux2/1 -> Bus Creator/2  "uprop"
  RPM2ManifoldPressure/1 -> Mux2/2
  flip sign3/1 -> Scope3/1, Bus Creator/1  "uaero"
  Mux1/1 -> flip sign3/1
  Look-Up Table/1 -> Mux1/4
  Rate Limiter/1 -> Look-Up Table/1
  Rudder/1 -> Sum/1
  Rudder Trim/1 -> Sum/2
  Flap/1 -> Rate Limiter/1

== system ap_12BAdapted_with_contracts_AutoPilot/ap_12BAdapted_AutopilotSpec/AP-000 ==
  In1 : Inport
  guarantee : Outport  OutDataTypeStr=boolean
  wires:
  In1/1 -> guarantee/1

== system ap_12BAdapted_with_contracts_AutoPilot/ap_12BAdapted_AutopilotSpec/AP-005 ==
  In1 : Inport
  guarantee : Outport  OutDataTypeStr=boolean
  wires:
  In1/1 -> guarantee/1

== system ap_12BAdapted_with_contracts_AutoPilot/ap_12BAdapted_AutopilotSpec/AP-006 ==
  In1 : Inport
  guarantee : Outport  OutDataTypeStr=boolean
  wires:
  In1/1 -> guarantee/1

== system ap_12BAdapted_with_contracts_AutoPilot/ap_12BAdapted_AutopilotSpec/abs_real_call ==
  abs_real_x : Inport  OutDataTypeStr=double
  branch_6_IF : Switch  Criteria=u2 ~= 0
  xxabs_real_1_operator : RelationalOperator  OutDataTypeStr=boolean  RndMeth=Simplest
  xxabs_real_1_rhs_2 : Constant  Value=0.0  OutDataTypeStr=double
  xxabs_real_2_operator : Gain  Gain=-1  OutDataTypeStr=double
  abs_real_y : Outport
  wires:
  branch_6_IF/1 -> abs_real_y/1
  xxabs_real_1_rhs_2/1 -> xxabs_real_1_operator/2
  xxabs_real_2_operator/1 -> branch_6_IF/3
  xxabs_real_1_operator/1 -> branch_6_IF/2
  abs_real_x/1 -> xxabs_real_2_operator/1, xxabs_real_1_operator/1, branch_6_IF/1

== system ap_12BAdapted_with_contracts_AutoPilot/ap_12BAdapted_AutopilotSpec/abs_real_call1 ==
  abs_real_x : Inport  OutDataTypeStr=double
  branch_6_IF : Switch  Criteria=u2 ~= 0
  xxabs_real_1_operator : RelationalOperator  OutDataTypeStr=boolean  RndMeth=Simplest
  xxabs_real_1_rhs_2 : Constant  Value=0.0  OutDataTypeStr=double
  xxabs_real_2_operator : Gain  Gain=-1  OutDataTypeStr=double
  abs_real_y : Outport
  wires:
  branch_6_IF/1 -> abs_real_y/1
  xxabs_real_1_rhs_2/1 -> xxabs_real_1_operator/2
  xxabs_real_2_operator/1 -> branch_6_IF/3
  xxabs_real_1_operator/1 -> branch_6_IF/2
  abs_real_x/1 -> xxabs_real_2_operator/1, xxabs_real_1_operator/1, branch_6_IF/1

== system ap_12BAdapted_with_contracts_AutoPilot/ap_12BAdapted_AutopilotSpec/abs_real_call11 ==
  abs_real_x : Inport  OutDataTypeStr=double
  branch_6_IF : Switch  Criteria=u2 ~= 0
  xxabs_real_1_operator : RelationalOperator  OutDataTypeStr=boolean  RndMeth=Simplest
  xxabs_real_1_rhs_2 : Constant  Value=0.0  OutDataTypeStr=double
  xxabs_real_2_operator : Gain  Gain=-1  OutDataTypeStr=double
  abs_real_y : Outport
  wires:
  branch_6_IF/1 -> abs_real_y/1
  xxabs_real_1_rhs_2/1 -> xxabs_real_1_operator/2
  xxabs_real_2_operator/1 -> branch_6_IF/3
  xxabs_real_1_operator/1 -> branch_6_IF/2
  abs_real_x/1 -> xxabs_real_2_operator/1, xxabs_real_1_operator/1, branch_6_IF/1

== system ap_12BAdapted_with_contracts_AutoPilot/ap_12BAdapted_AutopilotSpec/abs_real_call111 ==
  abs_real_x : Inport  OutDataTypeStr=double
  branch_6_IF : Switch  Criteria=u2 ~= 0
  xxabs_real_1_operator : RelationalOperator  OutDataTypeStr=boolean  RndMeth=Simplest
  xxabs_real_1_rhs_2 : Constant  Value=0.0  OutDataTypeStr=double
  xxabs_real_2_operator : Gain  Gain=-1  OutDataTypeStr=double
  abs_real_y : Outport
  wires:
  branch_6_IF/1 -> abs_real_y/1
  xxabs_real_1_rhs_2/1 -> xxabs_real_1_operator/2
  xxabs_real_2_operator/1 -> branch_6_IF/3
  xxabs_real_1_operator/1 -> branch_6_IF/2
  abs_real_x/1 -> xxabs_real_2_operator/1, xxabs_real_1_operator/1, branch_6_IF/1

== system ap_12BAdapted_with_contracts_AutoPilot/ap_12BAdapted_AutopilotSpec/abs_real_call1111 ==
  abs_real_x : Inport  OutDataTypeStr=double
  branch_6_IF : Switch  Criteria=u2 ~= 0
  xxabs_real_1_operator : RelationalOperator  OutDataTypeStr=boolean  RndMeth=Simplest
  xxabs_real_1_rhs_2 : Constant  Value=0.0  OutDataTypeStr=double
  xxabs_real_2_operator : Gain  Gain=-1  OutDataTypeStr=double
  abs_real_y : Outport
  wires:
  branch_6_IF/1 -> abs_real_y/1
  xxabs_real_1_rhs_2/1 -> xxabs_real_1_operator/2
  xxabs_real_2_operator/1 -> branch_6_IF/3
  xxabs_real_1_operator/1 -> branch_6_IF/2
  abs_real_x/1 -> xxabs_real_2_operator/1, xxabs_real_1_operator/1, branch_6_IF/1

== system ap_12BAdapted_with_contracts_AutoPilot/ap_12BAdapted_AutopilotSpec/abs_real_call11111 ==
  abs_real_x : Inport  OutDataTypeStr=double
  branch_6_IF : Switch  Criteria=u2 ~= 0
  xxabs_real_1_operator : RelationalOperator  OutDataTypeStr=boolean  RndMeth=Simplest
  xxabs_real_1_rhs_2 : Constant  Value=0.0  OutDataTypeStr=double
  xxabs_real_2_operator : Gain  Gain=-1  OutDataTypeStr=double
  abs_real_y : Outport
  wires:
  branch_6_IF/1 -> abs_real_y/1
  xxabs_real_1_rhs_2/1 -> xxabs_real_1_operator/2
  xxabs_real_2_operator/1 -> branch_6_IF/3
  xxabs_real_1_operator/1 -> branch_6_IF/2
  abs_real_x/1 -> xxabs_real_2_operator/1, xxabs_real_1_operator/1, branch_6_IF/1

== system ap_12BAdapted_with_contracts_AutoPilot/ap_12BAdapted_AutopilotSpec/abs_real_call111111 ==
  abs_real_x : Inport  OutDataTypeStr=double
  branch_6_IF : Switch  Criteria=u2 ~= 0
  xxabs_real_1_operator : RelationalOperator  OutDataTypeStr=boolean  RndMeth=Simplest
  xxabs_real_1_rhs_2 : Constant  Value=0.0  OutDataTypeStr=double
  xxabs_real_2_operator : Gain  Gain=-1  OutDataTypeStr=double
  abs_real_y : Outport
  wires:
  branch_6_IF/1 -> abs_real_y/1
  xxabs_real_1_rhs_2/1 -> xxabs_real_1_operator/2
  xxabs_real_2_operator/1 -> branch_6_IF/3
  xxabs_real_1_operator/1 -> branch_6_IF/2
  abs_real_x/1 -> xxabs_real_2_operator/1, xxabs_real_1_operator/1, branch_6_IF/1

== system ap_12BAdapted_with_contracts_AutoPilot/ap_12BAdapted_AutopilotSpec/hdg_mode ==
  note: Shouldn't not be edited
  require : Inport  OutDataTypeStr=boolean
  ensure : Inport  Port=2  OutDataTypeStr=boolean
  and : Logic  Operator=NOT  IconShape=distinctive  AllPortsSameDT=off  OutDataTypeStr=boolean
  or : Logic  Operator=OR  IconShape=distinctive  AllPortsSameDT=off  OutDataTypeStr=boolean
  mode : Outport
  wires:
  or/1 -> mode/1
  ensure/1 -> or/2
  and/1 -> or/1
  require/1 -> and/1

== system ap_12BAdapted_with_contracts_AutoPilot/ap_12BAdapted_AutopilotSpec/hdg_mode_ensure ==
  In1 : Inport
  ensure : Outport  OutDataTypeStr=boolean
  wires:
  In1/1 -> ensure/1

== system ap_12BAdapted_with_contracts_AutoPilot/ap_12BAdapted_AutopilotSpec/hdg_mode_require ==
  In1 : Inport
  require : Outport  OutDataTypeStr=boolean
  wires:
  In1/1 -> require/1

== system ap_12BAdapted_with_contracts_AutoPilot/ap_12BAdapted_AutopilotSpec/roll_hold_mode ==
  note: Shouldn't not be edited
  require : Inport  OutDataTypeStr=boolean
  ensure : Inport  Port=2  OutDataTypeStr=boolean
  and : Logic  Operator=NOT  IconShape=distinctive  AllPortsSameDT=off  OutDataTypeStr=boolean
  or : Logic  Operator=OR  IconShape=distinctive  AllPortsSameDT=off  OutDataTypeStr=boolean
  mode : Outport
  wires:
  or/1 -> mode/1
  ensure/1 -> or/2
  and/1 -> or/1
  require/1 -> and/1

== system ap_12BAdapted_with_contracts_AutoPilot/ap_12BAdapted_AutopilotSpec/roll_hold_mode_ensure ==
  In1 : Inport
  ensure : Outport  OutDataTypeStr=boolean
  wires:
  In1/1 -> ensure/1

== system ap_12BAdapted_with_contracts_AutoPilot/ap_12BAdapted_AutopilotSpec/roll_hold_mode_require ==
  In1 : Inport
  require : Outport  OutDataTypeStr=boolean
  wires:
  In1/1 -> require/1

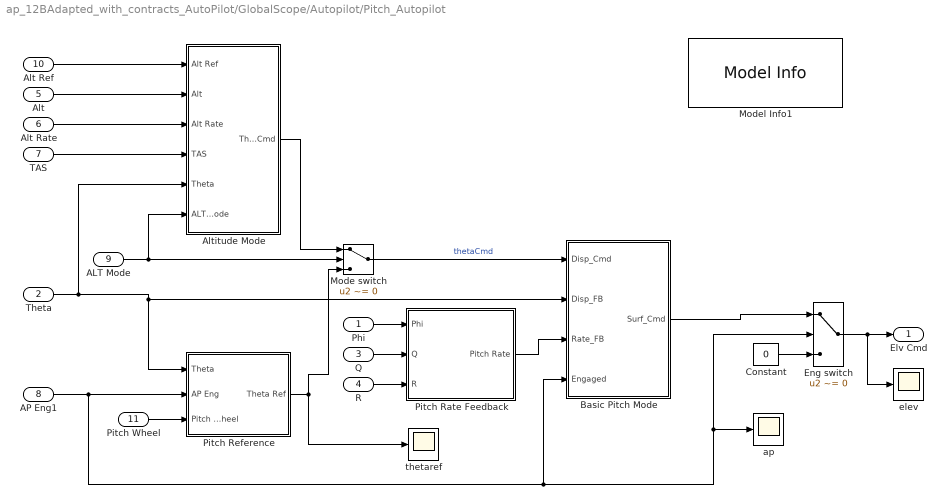
== system ap_12BAdapted_with_contracts_AutoPilot/GlobalScope/Autopilot/Pitch_Autopilot ==
  Phi : Inport  OutDataTypeStr=double  PortDimensions=1  SampleTime=1/40  Interpolate=off
  Theta : Inport  Port=2  OutDataTypeStr=double  PortDimensions=1  SampleTime=1/40  Interpolate=off
  Q : Inport  Port=3  OutDataTypeStr=double  PortDimensions=1  SampleTime=1/40  Interpolate=off
  R : Inport  Port=4  OutDataTypeStr=double  PortDimensions=1  SampleTime=1/40  Interpolate=off
  Alt : Inport  Port=5  OutDataTypeStr=double  PortDimensions=1  SampleTime=1/40  Interpolate=off
  Alt Rate : Inport  Port=6  OutDataTypeStr=double  PortDimensions=1  SampleTime=1/40  Interpolate=off
  TAS : Inport  Port=7  OutDataTypeStr=double  PortDimensions=1  SampleTime=1/40  Interpolate=off
  AP Eng1 : Inport  Port=8  OutDataTypeStr=boolean  PortDimensions=1  SampleTime=1/40  Interpolate=off
  ALT Mode : Inport  Port=9  OutDataTypeStr=boolean  PortDimensions=1  SampleTime=1/40  Interpolate=off
  Alt Ref : Inport  Port=10  OutDataTypeStr=double  PortDimensions=1  SampleTime=1/40  Interpolate=off
  "Pitch Wheel " : Inport  Port=11  OutDataTypeStr=double  PortDimensions=1  SampleTime=1/40  Interpolate=off
  Altitude Mode : Subsystem
  Basic Pitch Mode : Subsystem
  Constant : Constant  Value=0  OutDataTypeStr=double
  Eng switch : Switch  Criteria=u2 ~= 0
  Mode switch : Switch  Criteria=u2 ~= 0
  Model Info1 : simulink/Model-Wide Utilities/Model Info  Frame=on  DisplayStringWithTags=|  HorizontalTextAlignment=Left  LeftAlignmentValue=0.02
      | Pitch Autopilot
      | Author: %<LastModifiedBy>
      | Date: %<LastModificationDate>
      | Model Version: %<ModelVersion>
  Pitch Rate Feedback : Subsystem  TreatAsAtomicUnit=on
      settings: RTWSystemCode=Inline
  Pitch Reference : Subsystem  TreatAsAtomicUnit=on
      settings: RTWSystemCode=Inline
  ap : Scope
  elev : Scope
  thetaref : Scope
  Elv Cmd : Outport  OutDataTypeStr=double  PortDimensions=1  SampleTime=1/40  VectorParamsAs1DForOutWhenUnconnected=off
  wires:
  "Pitch Wheel "/1 -> Pitch Reference/3(Pitch Wheel)
  Pitch Rate Feedback/1(Pitch Rate) -> Basic Pitch Mode/3(Rate_FB)
  Alt Ref/1 -> Altitude Mode/1(Alt Ref)
  Theta/1 -> Altitude Mode/5(Theta), Pitch Reference/1(Theta), Basic Pitch Mode/2("Disp_FB ")
  Q/1 -> Pitch Rate Feedback/2(Q)
  Eng switch/1 -> elev/1, Elv Cmd/1
  Constant/1 -> Eng switch/3
  Phi/1 -> Pitch Rate Feedback/1(Phi)
  R/1 -> Pitch Rate Feedback/3(R)
  TAS/1 -> Altitude Mode/4(TAS)
  Pitch Reference/1(Theta Ref) -> thetaref/1, Mode switch/3
  Alt/1 -> Altitude Mode/2(Alt)
  Alt Rate/1 -> Altitude Mode/3(Alt Rate)
  Mode switch/1 -> Basic Pitch Mode/1(Disp_Cmd)  "thetaCmd"
  ALT Mode/1 -> Altitude Mode/6(ALT Mode), Mode switch/2
  Altitude Mode/1(Theta Cmd) -> Mode switch/1
  AP Eng1/1 -> Eng switch/2, ap/1, Basic Pitch Mode/4(Engaged), Pitch Reference/2(AP Eng)
  Basic Pitch Mode/1(Surf_Cmd) -> Eng switch/1

== system ap_12BAdapted_with_contracts_AutoPilot/GlobalScope/Autopilot/Roll_Autopilot ==
  Phi : Inport  OutMin=-180  OutMax=180  OutDataTypeStr=double  PortDimensions=1  SampleTime=1/40  Interpolate=off
  Psi : Inport  Port=2  OutMin=-180  OutMax=180  OutDataTypeStr=double  PortDimensions=1  SampleTime=1/40  Interpolate=off
  p : Inport  Port=3  OutMin=-180  OutMax=180  OutDataTypeStr=double  PortDimensions=1  Interpolate=off
  TAS : Inport  Port=4  OutMin=0  OutMax=1000  OutDataTypeStr=double  PortDimensions=1  SampleTime=1/40  Interpolate=off
  AP Eng : Inport  Port=5  OutDataTypeStr=boolean  PortDimensions=1  SampleTime=1/40  Interpolate=off
  HDG Mode : Inport  Port=6  OutDataTypeStr=boolean  PortDimensions=1  SampleTime=1/40  Interpolate=off
  HDG Ref : Inport  Port=7  OutMin=-180  OutMax=180  OutDataTypeStr=double  PortDimensions=1  SampleTime=1/40  Interpolate=off
  Turn Knob : Inport  Port=8  OutMin=-45  OutMax=45  OutDataTypeStr=double  PortDimensions=1  SampleTime=1/40  Interpolate=off
  Basic Roll Mode : Subsystem
  Eng switch : Switch  Criteria=u2 ~= 0
  Heading Mode : Subsystem
  Mode switch : Switch  Criteria=u2 ~= 0
  Roll Reference : Subsystem  TreatAsAtomicUnit=on
      settings: RTWSystemCode=Inline
  Scope1 : Scope
  zero : Constant  Value=0  OutDataTypeStr=double
  Ail Cmd : Outport  OutDataTypeStr=double  PortDimensions=1  SampleTime=1/40  VectorParamsAs1DForOutWhenUnconnected=off
  HdgMode_cmd : Outport  Port=2  VectorParamsAs1DForOutWhenUnconnected=off
  PhiRef_cmd : Outport  Port=3  VectorParamsAs1DForOutWhenUnconnected=off
  phiCmd : Outport  Port=4  VectorParamsAs1DForOutWhenUnconnected=off
  wires:
  HDG Ref/1 -> Heading Mode/1(Psi Ref)
  Heading Mode/1(Phi Cmd) -> HdgMode_cmd/1, Mode switch/1
  Mode switch/1 -> phiCmd/1, Basic Roll Mode/1(Disp_Cmd)  "phiCmd"
  Eng switch/1 -> Ail Cmd/1
  AP Eng/1 -> Roll Reference/2(AP eng), Basic Roll Mode/4(Engaged), Eng switch/2
  TAS/1 -> Heading Mode/3(TAS)
  HDG Mode/1 -> Mode switch/2
  Roll Reference/1(Phi Ref) -> Mode switch/3, PhiRef_cmd/1
  Turn Knob/1 -> Roll Reference/3(Turn Knob)
  zero/1 -> Eng switch/3
  p/1 -> Basic Roll Mode/3(Rate_FB)
  Phi/1 -> Scope1/1, Basic Roll Mode/2("Disp_FB "), Roll Reference/1(Phi)
  Psi/1 -> Heading Mode/2(Psi)
  Basic Roll Mode/1(Surf_Cmd) -> Eng switch/1

== system ap_12BAdapted_with_contracts_AutoPilot/GlobalScope/Autopilot/Yaw_damper ==
  Phi : Inport  OutDataTypeStr=double  PortDimensions=1  SampleTime=1/40  Interpolate=off
  R : Inport  Port=2  OutDataTypeStr=double  PortDimensions=1  SampleTime=1/40  Interpolate=off
  TAS : Inport  Port=3  OutDataTypeStr=double  PortDimensions=1  SampleTime=1/40  Interpolate=off
  AP Eng : Inport  Port=4  OutDataTypeStr=boolean  PortDimensions=1  SampleTime=1/40  Interpolate=off
  Basic Yaw Damper : Subsystem  TreatAsAtomicUnit=on
      settings: RTWSystemCode=Inline
  Constant : Constant  Value=0  OutDataTypeStr=double
  Eng switch : Switch  Criteria=u2 ~= 0
  Model Info1 : simulink/Model-Wide Utilities/Model Info  Frame=on  DisplayStringWithTags=|  HorizontalTextAlignment=Left  LeftAlignmentValue=0.02
      | Yaw Damper
      | Author: %<LastModifiedBy>
      | Version: %<ModelVersion>
      | Date: %<LastModificationDate>
  Rud Cmd : Outport  OutDataTypeStr=double  PortDimensions=1  SampleTime=1/40  VectorParamsAs1DForOutWhenUnconnected=off
  wires:
  Phi/1 -> Basic Yaw Damper/1("Phi ")
  R/1 -> Basic Yaw Damper/2(R)
  Constant/1 -> Eng switch/3
  TAS/1 -> Basic Yaw Damper/3(TAS)
  Basic Yaw Damper/1(Rud Cmd) -> Eng switch/1
  Eng switch/1 -> Rud Cmd/1
  AP Eng/1 -> Eng switch/2

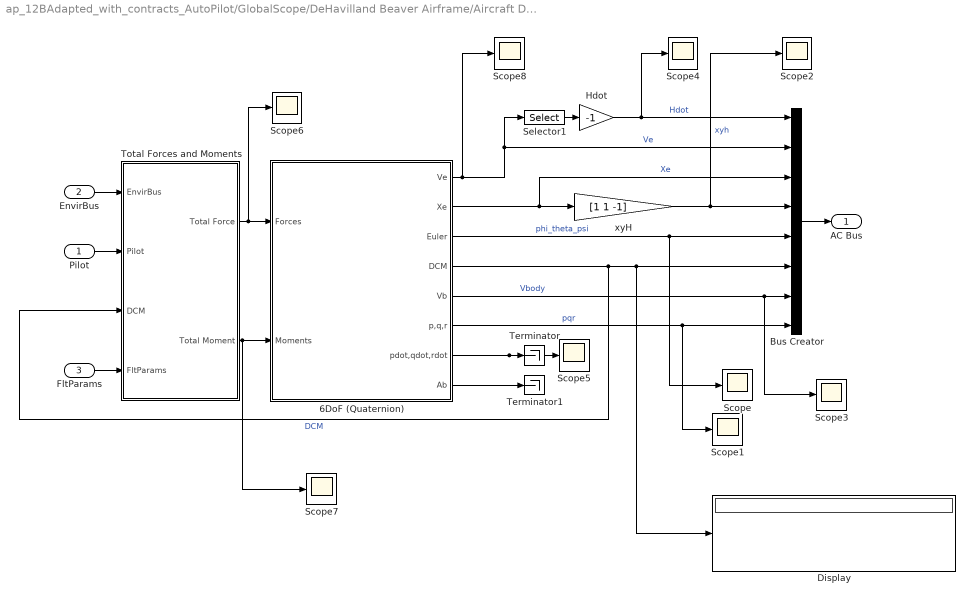
== system ap_12BAdapted_with_contracts_AutoPilot/GlobalScope/DeHavilland Beaver Airframe/Aircraft Dynamics ==
  Pilot : Inport
  EnvirBus : Inport  Port=2
  FltParams : Inport  Port=3
  6DoF (Quaternion) : Subsystem
  Bus Creator : BusCreator  Inputs=8
  Display : Display
  Hdot : Gain  Gain=-1  SaturateOnIntegerOverflow=on  OutDataTypeStr=Inherit: Same as input  ParamDataTypeStr=Inherit: Same as input
  Scope{,1..8} (9 alike) : Scope
  Selector1 : Selector  InputPortWidth=3  IndexOptions=Index vector (dialog)  Indices=[3]  OutputSizes=1
  Terminator : Terminator
  Terminator1 : Terminator
  Total Forces and Moments : Subsystem
  xyH : Gain  Gain=[1 1 -1]  SaturateOnIntegerOverflow=on  OutDataTypeStr=Inherit: Same as input  ParamDataTypeStr=Inherit: Same as input
  AC Bus : Outport  VectorParamsAs1DForOutWhenUnconnected=off
  wires:
  6DoF (Quaternion)/4(DCM) -> Display/1, Bus Creator/6, Total Forces and Moments/3(DCM)  "DCM"
  6DoF (Quaternion)/3(Euler) -> Scope/1, Bus Creator/5  "phi_theta_psi"
  6DoF (Quaternion)/2(Xe) -> xyH/1, Bus Creator/3  "Xe"
  6DoF (Quaternion)/5(Vb) -> Scope3/1, Bus Creator/7  "Vbody"
  6DoF (Quaternion)/7(pdot,qdot,rdot) -> Scope5/1, Terminator/1
  6DoF (Quaternion)/1(Ve) -> Scope8/1, Selector1/1, Bus Creator/2  "Ve"
  Pilot/1 -> Total Forces and Moments/2(Pilot)
  Selector1/1 -> Hdot/1
  Total Forces and Moments/1(Total Force) -> Scope6/1, 6DoF (Quaternion)/1(Forces)
  Total Forces and Moments/2(Total Moment) -> Scope7/1, 6DoF (Quaternion)/2(Moments)
  xyH/1 -> Scope2/1, Bus Creator/4  "xyh"
  Hdot/1 -> Scope4/1, Bus Creator/1  "Hdot"
  6DoF (Quaternion)/8(Ab) -> Terminator1/1
  Bus Creator/1 -> AC Bus/1
  EnvirBus/1 -> Total Forces and Moments/1(EnvirBus)
  6DoF (Quaternion)/6(p,q,r) -> Scope1/1, Bus Creator/8  "pqr"
  FltParams/1 -> Total Forces and Moments/4(FltParams)

== system ap_12BAdapted_with_contracts_AutoPilot/GlobalScope/DeHavilland Beaver Airframe/Calculate Parameters ==
  EnvirBus : Inport
  ACBus : Inport  Port=2
  " Incidence, Sideslip, & Airspeed" : Subsystem
  "ACBus " : InportShadow  Port=2
  Bus Creator : BusCreator  Inputs=5
  Bus Selector1 : BusSelector  OutputSignals=rho
  Bus Selector2 : BusSelector  OutputSignals=Vbody
  Bus Selector3 : BusSelector  OutputSignals=pqr,Ve
  Bus Selector4 : BusSelector  OutputSignals=Vwind.uvw_wind,Vwind.pqr_wind
  Display : Display
  Dynamic Pressure : Subsystem
  Scope{,1..5} (6 alike) : Scope
  Sum2 : Sum  Inputs=|++  SaturateOnIntegerOverflow=on  InputSameDT=on  OutDataTypeStr=Inherit: Same as first input
  Sum4 : Sum  Inputs=+-|  SaturateOnIntegerOverflow=on  InputSameDT=on  OutDataTypeStr=Inherit: Same as first input
  FltParams : Outport  VectorParamsAs1DForOutWhenUnconnected=off
  wires:
  "ACBus "/1 -> Bus Selector2/1
  Bus Creator/1 -> Scope/1, FltParams/1
  Bus Selector3/1 -> Scope3/1, Sum2/2  "<pqr>"
  ACBus/1 -> Bus Selector3/1
  Bus Selector1/1 -> Scope4/1, Dynamic Pressure/2(Air Density)  "<rho>"
  EnvirBus/1 -> Bus Selector1/1, Bus Selector4/1
  Dynamic Pressure/1(qbar) -> Display/1, Bus Creator/5  "Qdyn"
  Bus Selector3/2 -> Scope5/1, Dynamic Pressure/1(Velocity)  "<Ve>"
  Bus Selector4/2 -> Sum2/1  "<pqr_wind>"
  Sum4/1 -> " Incidence, Sideslip, & Airspeed"/1(Vb)
  " Incidence, Sideslip, & Airspeed"/1(Alpha) -> Scope1/1, Bus Creator/1  "alpha"
  " Incidence, Sideslip, & Airspeed"/2(Beta) -> Bus Creator/2  "beta"
  " Incidence, Sideslip, & Airspeed"/3(V) -> Bus Creator/3  "V"
  Bus Selector2/1 -> Scope2/1, Sum4/1  "<Vbody>"
  Bus Selector4/1 -> Sum4/2  "<uvw_wind>"
  Sum2/1 -> Bus Creator/4  "pqr_tot"

== system ap_12BAdapted_with_contracts_AutoPilot/GlobalScope/Sensors/Air Data Sensor ==
  note: Air Data Sensor
  AC Bus : Inport
  " Incidence, Sideslip, & Airspeed" : Subsystem
  Bus Selector1 : BusSelector  OutputSignals=Hdot,Vbody,xyh
  Constant1 : Constant  Value=trim_v
  Constant2 : Constant  Value=0.0
  Constant3 : Constant  Value=trim_altref
  Selector1 : Selector  InputPortWidth=3  IndexOptions=Index vector (dialog)  Indices=[3]  OutputSizes=1
  flip sign1 : Gain  Gain=m2ft  SaturateOnIntegerOverflow=on  OutDataTypeStr=Inherit: Same as input  ParamDataTypeStr=Inherit: Same as input
  flip sign2 : Gain  Gain=m2ft  SaturateOnIntegerOverflow=on  OutDataTypeStr=Inherit: Same as input  ParamDataTypeStr=Inherit: Same as input
  flip sign3 : Gain  Gain=m2ft  SaturateOnIntegerOverflow=on  OutDataTypeStr=Inherit: Same as input  ParamDataTypeStr=Inherit: Same as input
  ic1 : Subsystem
  ic2 : Subsystem
  ic3 : Subsystem
  altRate : Outport  VectorParamsAs1DForOutWhenUnconnected=off
  alpha : Outport  Port=2  VectorParamsAs1DForOutWhenUnconnected=off
  beta : Outport  Port=3  VectorParamsAs1DForOutWhenUnconnected=off
  airspeed : Outport  Port=4  VectorParamsAs1DForOutWhenUnconnected=off
  alt : Outport  Port=5  VectorParamsAs1DForOutWhenUnconnected=off
  wires:
  Constant1/1 -> ic1/2(ic)
  AC Bus/1 -> Bus Selector1/1
  flip sign3/1 -> ic2/1(u)  "alt"
  " Incidence, Sideslip, & Airspeed"/2(Beta) -> beta/1  "beta"
  Selector1/1 -> flip sign3/1
  ic1/1(y) -> flip sign1/1
  Constant3/1 -> ic2/2(ic)
  Constant2/1 -> ic3/2(ic)
  Bus Selector1/2 -> ic1/1(u)  "<Vbody>"
  " Incidence, Sideslip, & Airspeed"/3(V) -> airspeed/1  "airspeed"
  " Incidence, Sideslip, & Airspeed"/1(Alpha) -> alpha/1  "alpha"
  Bus Selector1/3 -> Selector1/1  "<xyh>"
  flip sign2/1 -> ic3/1(u)  "Hdotfps"
  ic2/1(y) -> alt/1  "alt"
  Bus Selector1/1 -> flip sign2/1  "<Hdot>"
  ic3/1(y) -> altRate/1  "altRate"
  flip sign1/1 -> " Incidence, Sideslip, & Airspeed"/1(Vb)  "Vfps"
